simulink model "ampc_cstr_linearization"  (R2021a)
settings: Solver=VariableStepAuto  StartTime=0.0  StopTime=400  MaxStep=0.5  RelTol=1e-3
undefined symbols (not defined in the file or in its folder): sigbuilder_block
libraries: mpclib x1, simulink x1
settings Model: Creator=NIFEMI  LastModifiedBy=USER
settings DataIOCC: ReturnWorkspaceOutputs=off
settings DebuggingCC: PregeneratedLibrarySubsystemCodeDiagnostic=none  SFMachineParentedDataDiag=warning  ArithmeticOperatorsInVariantConditions=warning
settings SFSimCC: CustomCodeUndefinedFunction=UseInterfaceOnly

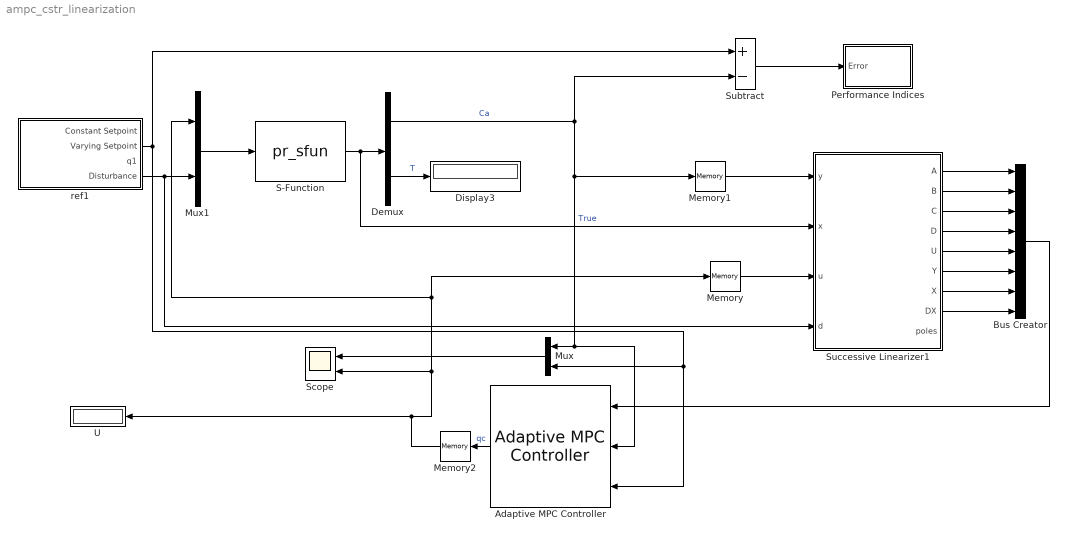
== system ampc_cstr_linearization ==
  Adaptive MPC Controller : mpclib/Adaptive MPC Controller  SCDEnableBlockLinearizationSpecification=on  mpcobj=mpcobj_sl  enable_value=0  updateMPCinCallerWorkspace=on  md_inport=off  mv_inport=off  uref_inport=off  return_cost=off  return_mvseq=off  return_qpstatus=off  return_xseq=off  return_state=off  return_ovseq=off  state_inport=off  isltv_plant=off  umin_inport=off  umax_inport=off  ymin_inport=off  ymax_inport=off  cc_inport=off  ywt_inport=off  uwt_inport=off  duwt_inport=off  rhoeps_inport=off  pm_inport=off  MaximumP=10  HorizonChoice=FixedHorizon  BlockDataType=double  SampleTimeInherited=off  switch_inport=off
  Bus Creator : BusCreator  Inputs=8
  Demux : Demux  Outputs=2
  Display3 : Display
  Memory : Memory  InitialCondition=103.41
  Memory1 : Memory  InitialCondition=0.1
  Memory2 : Memory  InitialCondition=103.41
  Mux : Mux  Inputs=2
  Mux1 : Mux  Inputs=2
  Performance Indices : Subsystem
  S-Function : S-Function  FunctionName=pr_sfun  SFunctionDeploymentMode=off  EnableBusSupport=off
  Scope : Scope  NumInputPorts=2
  Subtract : Sum  Inputs=+-
  Successive Linearizer1 : MATLAB Function  TreatAsAtomicUnit=on  SystemSampleTime=0.5
  U : Display
  "ref1 " : Subsystem  Tag=STV Subsys  LoadFcn=sigbuilder_block('load');  StartFcn=sigbuilder_block('start');  StopFcn=sigbuilder_block('stop');  ClipboardFcn=sigbuilder_block('clipboard');  mask(Sigbuilder block){tuvar=[0:10]}
      mask help: Simulink:masks:SigbuilderBlock_MD
      mask init:
      | if ~strcmp(get_param(bdroot(gcbh),'SimulationStatus'),'stopped') tuvar = sigbuilder_block('maskInit'); end
      settings: CopyFcn=sigbuilder_block('copy');  DeleteFcn=sigbuilder_block('delete');  ModelCloseFcn=sigbuilder_block('modelClose');  PreSaveFcn=sigbuilder_block('preSave');  PauseFcn=sigbuilder_block('pause');  ContinueFcn=sigbuilder_block('continue');  NameChangeFcn=sigbuilder_block('namechange');  OpenFcn=sigbuilder_block('open',[5.5 0 949 448 ]);  CloseFcn=sigbuilder_block('close');
      mask Display: plot(0, 0, 100, 100,[2, 2, 32, 32, 2], [68, 8, 8, 68, 68],[32, 2], [38, 38], [32, 19, 2],[53, 60, 44], [32, 17, 17, 2],[16, 16, 31, 31]);txt = getActiveGroup(gcbh);text(2, 100, txt,'verticalAlignment', 'top');
  wires:
  Successive Linearizer1/1(A) -> Bus Creator/1
  Successive Linearizer1/2(B) -> Bus Creator/2
  Successive Linearizer1/3(C) -> Bus Creator/3
  Successive Linearizer1/5(U) -> Bus Creator/5
  Successive Linearizer1/6(Y) -> Bus Creator/6
  Successive Linearizer1/7(X) -> Bus Creator/7
  Successive Linearizer1/8(DX) -> Bus Creator/8
  Successive Linearizer1/4(D) -> Bus Creator/4
  Bus Creator/1 -> Adaptive MPC Controller/1
  Mux/1 -> Scope/1
  Subtract/1 -> Performance Indices/1(Error)
  "ref1 "/2(Varying Setpoint) -> Subtract/1, Adaptive MPC Controller/3, Mux/2
  Adaptive MPC Controller/1 -> Memory2/1  "qc"
  S-Function/1 -> Successive Linearizer1/2(x), Demux/1  "True"
  Demux/1 -> Adaptive MPC Controller/2, Mux/1, Memory1/1, Subtract/2  "Ca"
  Mux1/1 -> S-Function/1
  "ref1 "/4(Disturbance) -> Successive Linearizer1/4(d), Mux1/2
  Demux/2 -> Display3/1  "T"
  Memory1/1 -> Successive Linearizer1/1(y)
  Memory/1 -> Successive Linearizer1/3(u)
  Memory2/1 -> Memory/1, Mux1/1, Scope/2, U/1

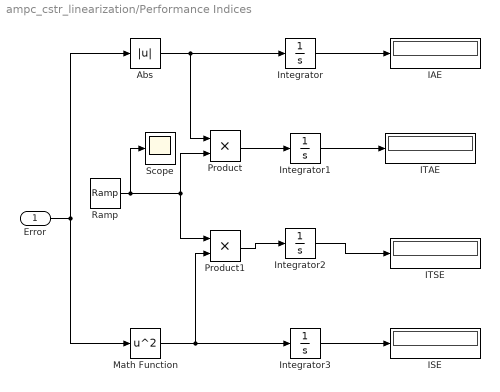
== system ampc_cstr_linearization/Performance Indices ==
  Error : Inport
  Abs : Abs
  IAE : Display
  ISE : Display
  ITAE : Display
  ITSE : Display
  Integrator{,1..3} (4 alike) : Integrator
  Math Function : Math  Operator=square  SignedPower=on  SaturateOnIntegerOverflow=on
  Product : Product  RndMeth=Zero
  Product1 : Product  RndMeth=Zero
  Ramp : simulink/Sources/Ramp  slope=1  start=0  InitialOutput=0
  Scope : Scope
  wires:
  Error/1 -> Math Function/1, Abs/1
  Abs/1 -> Integrator/1, Product/1
  Integrator/1 -> IAE/1
  Ramp/1 -> Product/2, Product1/1, Scope/1
  Math Function/1 -> Integrator3/1, Product1/2
  Product1/1 -> Integrator2/1
  Product/1 -> Integrator1/1
  Integrator3/1 -> ISE/1
  Integrator2/1 -> ITSE/1
  Integrator1/1 -> ITAE/1

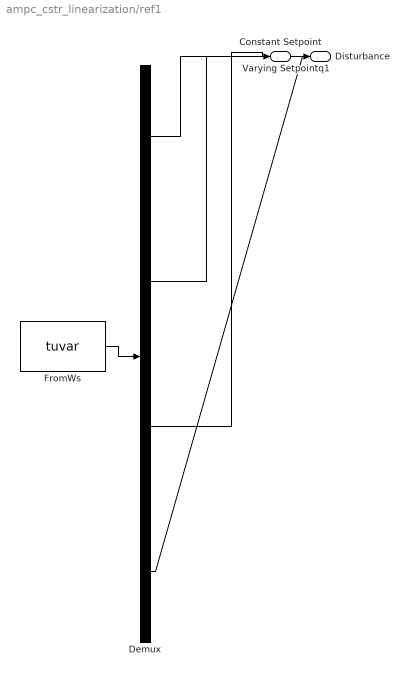
== system ampc_cstr_linearization/ref1  ==
  Demux : Demux  Tag=STV Demux
      settings: DisplayOption=none
  FromWs : FromWorkspace  Tag=STV FromWs  VariableName=tuvar
      SigBuilderData=|
      | common.afterFinalStr = 'Extrapolate'
      | common.sampleTime = 0
      | dataSet.timeRange = [0 400]
      | dataSet.name = 'Group 1'
      | sbobj.Groups.Name = 'Group 1'
      | sbobj.Groups.Signals(1).Name = 'Constant Setpoint'
      | sbobj.Groups.Signals(1).XData = [0 400]
      | sbobj.Groups.Signals(1).YData = [0.1 0.1]
      | sbobj.Groups.Signals(2).Name = 'Varying Setpoint'
      | sbobj.Groups.Signals(2).XData = [0 50 50 150 150 300 300 400]
      | sbobj.Groups.Signals(2).YData = [0.085 0.085 0.1 0.1 0.04 0.04 0.1 0.1]
      | sbobj.Groups.Signals(3).Name = 'q1'
      | sbobj.Groups.Signals(3).XData = [0 400]
      | sbobj.Groups.Signals(3).YData = [100 100]
      | sbobj.Groups.Signals(4).Name = 'Disturbance'
      | sbobj.Groups.Signals(4).XData = [0 50 50 150 150 300 300 400]
      | sbobj.Groups.Signals(4).YData = [100 100 95 95 105 105 100 100]
      | sbobj.Groups.TimeRange = [0 400]
  Constant Setpoint : Outport  Tag=STV Outport
  Varying Setpoint : Outport  Tag=STV Outport  Port=2  VectorParamsAs1DForOutWhenUnconnected=off
  q1 : Outport  Tag=STV Outport  Port=3
  Disturbance : Outport  Tag=STV Outport  Port=4
  wires:
  FromWs/1 -> Demux/1
  Demux/1 -> Constant Setpoint/1
  Demux/2 -> Varying Setpoint/1
  Demux/3 -> q1/1
  Demux/4 -> Disturbance/1

== matlab function ampc_cstr_linearization/Successive Linearizer1 ==
  data: y input size=[1,1]; x input; A output size=[2,2]; B output size=[2 1]; C output size=[1,2]; D output size=[1 1]; U output size=[1,1]; Y output size=[1,1]; X output size=[2,1]; DX output size=[2,1]; u input; d input; poles output
function [A, B, C, D, U, Y, X, DX,poles] = fcn(y, x, u, d)

%%%%%%%%%%%%%%%%%%%%%%%%%%%%%%%%%%%%%%%%%%%%%%%%%%%%%%%
%#codegen

% Define constant outputs
Ts = 0.1;
U = u(1) ;
Y = y ;
X = x(1:2) ;



% Analytical linearization of mechanistic CSTR model (continuous time)
% [A, Bo] = getContinuous(T, CA, CAi, Ti, Tc);
[a, b, c, d] = getContinuous(y, x, u, d, Ts)  ;

% Convert continuous to discrete time
% [A, Bo] = getDiscrete(A, Bo, Ts);
[A, Bo, C, D] = getDiscrete(a, b, c, d, Ts)   ;
% Last column of B contains the constant offset contribution.
DX = Bo(:,2);
B = Bo(:,1);
% Compute poles
poles = abs(eig(A));

end

%%%%%%%%%%%%%%%%%%%%%%%%%%%%%%%%%%%%%%%%%%%%%%%%%%%%%
%%%%%%%%%%%%%%%%%%%%%%%%%%%%%%%%%%%

function [a, b, c, d] = getContinuous(y, x, u, d, Ts)




% [A, B, C, D] = get_discrete_model(y, x, u, d, Ts)   ;

%%%%%%%%%%%%%%%%%%%%%%%%%%%%%%%%%%%%%   
qc = u(1);
q = d(1);

x_1 = x(1);
x_2 = x(2);
    
Ca0 = 1;
T0 = 350;
Tc0 = 350;
v = 100;
HA = 7e5;
k = 7.2e10;
E_R = 1e4;
deltaH = -2e5;
rho = 1e3;
rho_c = 1e3;
cp = 1;
cpc = 1;
      
dx_1dt = ((q/v)*(Ca0 - x_1)) - (k*x_1*exp(-E_R/x_2)); 
dx_2dt = ((q/v)*(T0 - x_2)) - (((deltaH*k*x_1)/(rho*cp))*exp(-E_R/x_2)) + ((rho_c*cpc)/(rho*cp*v))*qc*(1- exp(-HA/(qc*rho*cp)))*(Tc0-x_2);
%dx_2dt = (q/v)*(T0 - x_2) - ((deltaH*k*x_1)/(rho*cp))*exp((-E_R)*(1/x_2))+((rho_c*cpc)/(rho*cp*v))*qc*(1-exp((-HA)/(qc*rho*cp)))*(Tc0-x_2);
      
%dxdt = [dx_1dt; dx_2dt];
%%%%%%%%%%%%%%%%%%%%%%%%%%%%%%%%%%  
qc = u(1);
q = d(1);
Ca0 = 1;
T0 = 350;


x_1 = x(1);
x_2 = x(2);
       
Ca = y(1);
 
a = [ - q/100 - 72000000000*exp(-10000/x_2),                                     -(720000000000000*x_1*exp(-10000/x_2))/x_2^2;
        -144000000000*exp(-10000/x_2), (qc*(exp(-7/qc) - 1))/100 - q/100 - (1440000000000000*x_1*exp(-10000/x_2))/x_2^2];

b =  [0 dx_1dt; ((x_2 - 350)*(exp(-7/qc) - 1))/100 + (7*exp(-7/qc)*(x_2 - 350))/(100*qc) dx_2dt];

c = [1,0];

d = 0;
    
  
    
    %%%%%%%%%%%%%%%%%%%%%%%%%%%%%%
    
       

end


function [A, B, C, D] = getDiscrete(a, b,c,d, Ts)
% Convert to discrete time
A = expm(a*Ts);
nx = size(b,1);
n = 4;  % Number of points for Simpson's Rule, an even integer >= 2.
% Use Simpson's rule to compute integral(0,Ts){expm(a*s)*ds*b}
h = Ts/n;
Ai = eye(nx) + A;        % First and last terms;
Coef = 2;
for i = 1:n-1
    if Coef == 2
        Coef = 4;
    else
        Coef = 2;
    end
    Ai = Ai + Coef*expm(a*i*h);     % Intermediate terms
end
B = (h/3)*Ai*b;

C = c  ;
D = d ;

end
